simulink model "Lab1_block_diagram"  (R2021a)
settings: Solver=VariableStepAuto  StartTime=0.0  StopTime=t  MaxStep=1e-3  RelTol=1e-3
undefined symbols (not defined in the file): A_1, A_2, b1, b2, b3, I1, I2, k1, k2, k3, T_1, T_2, x1_0, x2_0
settings Model: Creator=User  LastModifiedBy=User
settings SolverCC: SolverResetMethod=Robust

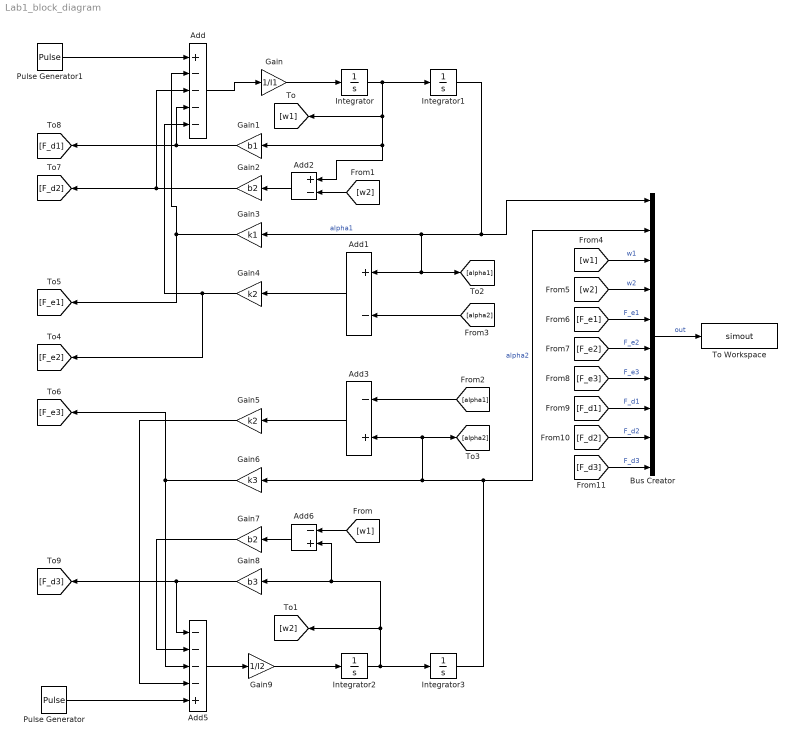
== system Lab1_block_diagram ==
  Add : Sum  Inputs=+----
  Add1 : Sum  Inputs=+-
  Add2 : Sum  Inputs=+-
  Add3 : Sum  Inputs=-+
  Add5 : Sum  Inputs=----+
  Add6 : Sum  Inputs=-+
  Bus Creator : BusCreator  Inputs=10
  Gain : Gain  Gain=1/I1
  Gain1 : Gain  Gain=b1
  Gain2 : Gain  Gain=b2
  Gain3 : Gain  Gain=k1
  Gain4 : Gain  Gain=k2
  Gain5 : Gain  Gain=k2
  Gain6 : Gain  Gain=k3
  Gain7 : Gain  Gain=b2
  Gain8 : Gain  Gain=b3
  Gain9 : Gain  Gain=1/I2
  Integrator : Integrator
  Integrator1 : Integrator  InitialCondition=x1_0
  Integrator2 : Integrator
  Integrator3 : Integrator  InitialCondition=x2_0
  Pulse Generator : DiscretePulseGenerator  PulseType=Time based  Amplitude=A_2  Period=T_2  PulseWidth=(0.5/T_2) * 100
  Pulse Generator1 : DiscretePulseGenerator  PulseType=Time based  Amplitude=A_1  Period=T_1  PulseWidth=(0.5/T_1) * 100
  To Workspace : ToWorkspace  VariableName=simout  SaveFormat=Timeseries  SampleTime=-1
  wires:
  Integrator/1 -> Add2/1, Gain1/1, [w1], Integrator1/1
  Gain/1 -> Integrator/1
  Add/1 -> Gain/1
  Add2/1 -> Gain2/1
  Add3/1 -> Gain5/1
  Add5/1 -> Gain9/1
  Gain9/1 -> Integrator2/1
  Integrator2/1 -> Add6/2, Gain8/1, [w2], Integrator3/1
  Add6/1 -> Gain7/1
  [w1] -> Add6/1
  [w2] -> Add2/2
  Add1/1 -> Gain4/1
  [alpha1] -> Add3/1
  [alpha2] -> Add1/2
  Gain1/1 -> [F_d1], Add/4
  Gain2/1 -> [F_d2], Add/3
  Gain3/1 -> [F_e1], Add/2
  Gain4/1 -> Add/5, [F_e2]
  Gain8/1 -> [F_d3], Add5/1
  Gain7/1 -> Add5/2
  Gain6/1 -> [F_e3], Add5/3
  Gain5/1 -> Add5/4
  Bus Creator/1 -> To Workspace/1  "out"
  Integrator1/1 -> Gain3/1, [alpha1], Add1/1, Bus Creator/1  "alpha1"
  Integrator3/1 -> Bus Creator/2, Gain6/1, [alpha2], Add3/2  "alpha2"
  [F_e1] -> Bus Creator/5  "F_e1"
  [F_e2] -> Bus Creator/6  "F_e2"
  [F_e3] -> Bus Creator/7  "F_e3"
  [F_d1] -> Bus Creator/8  "F_d1"
  [F_d2] -> Bus Creator/9  "F_d2"
  [F_d3] -> Bus Creator/10  "F_d3"
  [w2] -> Bus Creator/4  "w2"
  [w1] -> Bus Creator/3  "w1"
  Pulse Generator/1 -> Add5/5
  Pulse Generator1/1 -> Add/1
